simulink model "sig_kadet"  (R2022a)
settings: Solver=FixedStepAuto  StartTime=0.0  StopTime=10.0  FixedStep=framePeriod_s  RelTol=1e-3
undefined symbols (not defined in the file): Control, DiscIntNeverNeededParam, framePeriod_s
libraries: slpidlib x10, aerolibconvert2 x7, simulink_extras x2
(part 1 of 2)
settings Model: Creator=brian  LastModifiedBy=HP
settings SolverCC: AlgebraicLoopSolver=TrustRegion
settings OptimizationCC: DefaultParameterBehavior=Inlined  GainParamInheritBuiltInType=on  UseFloatMulNetSlope=on  DefaultUnderspecifiedDataType=single  InlineInvariantSignals=on  PassReuseOutputArgsAs=Individual arguments  ZeroExternalMemoryAtStartup=off  ZeroInternalMemoryAtStartup=off  NoFixptDivByZeroProtection=on  EfficientFloat2IntCast=on  LifeSpan=1  OptimizeBlockOrder=speed  DifferentSizesBufferReuse=on  EfficientTunableParamExpr=on
settings DebuggingCC: ParameterTunabilityLossMsg=error  UnconnectedInputMsg=warning  UnconnectedOutputMsg=warning  UnconnectedLineMsg=warning
settings HardwareCC: ProdBitPerPointer=32  ProdBitPerSizeT=32  ProdBitPerPtrDiffT=32  ProdLargestAtomicInteger=Long  ProdLargestAtomicFloat=Double  ProdWordSize=32  ProdLongLongMode=on  ProdHWDeviceType=NXP->Cortex-M4
settings ModelReferenceCC: ModelReferenceNumInstancesAllowed=Single
settings SFSimCC: SimParseCustomCode=off  MATLABDynamicMemAlloc=off
settings RTWCC: SystemTargetFile=ert.tlc  GenCodeOnly=on  TemplateMakefile=ert_default_tmf  RTWVerbose=off  Toolchain=Microsoft Visual C++ 2022 v17.0 | nmake (64-bit Windows)  BuildConfiguration=Faster Runs  TargetLang=C++  DLArmComputeVersion=19.05
settings CodeAppCC: ForceParamTrailComments=on  IgnoreCustomStorageClasses=off  OperatorAnnotations=on  SimulinkDataObjDesc=on  SFDataObjDesc=on  CustomSymbolStrGlobalVar=rt$N$M  CustomSymbolStrType=$N$M  CustomSymbolStrFcn=$N$M$F  CustomSymbolStrMacro=$N$M  InsertBlockDesc=on
settings ERTTargetCC: TargetLangStandard=C++03 (ISO)  IncludeMdlTerminateFcn=off  CombineSignalStateStructs=on  SuppressErrorStatus=on  SupportAbsoluteTime=off  CodeInterfacePackaging=C++ class  SupportNonFinite=off  SupportComplex=off  ERTHeaderFileRootName=autocode$E  ERTSourceFileRootName=autocode$E  InlinedParameterPlacement=NonHierarchical  RootIOFormat=Structure reference  ERTCustomFileTemplate=example_file_process.tlc  ERTFilePackagingFormat=Compact  ArrayContainerType=std::array

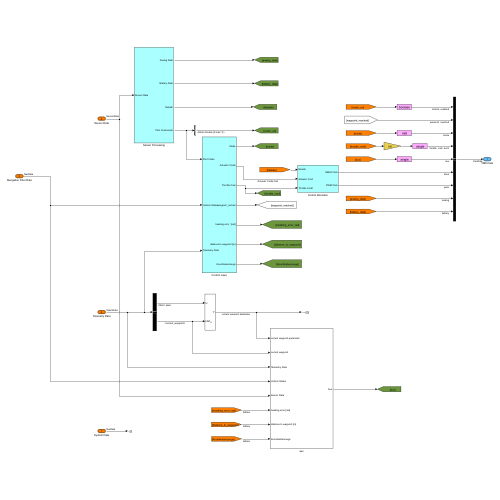
[thumbnail: Simulink's stored preview of the top-level diagram]
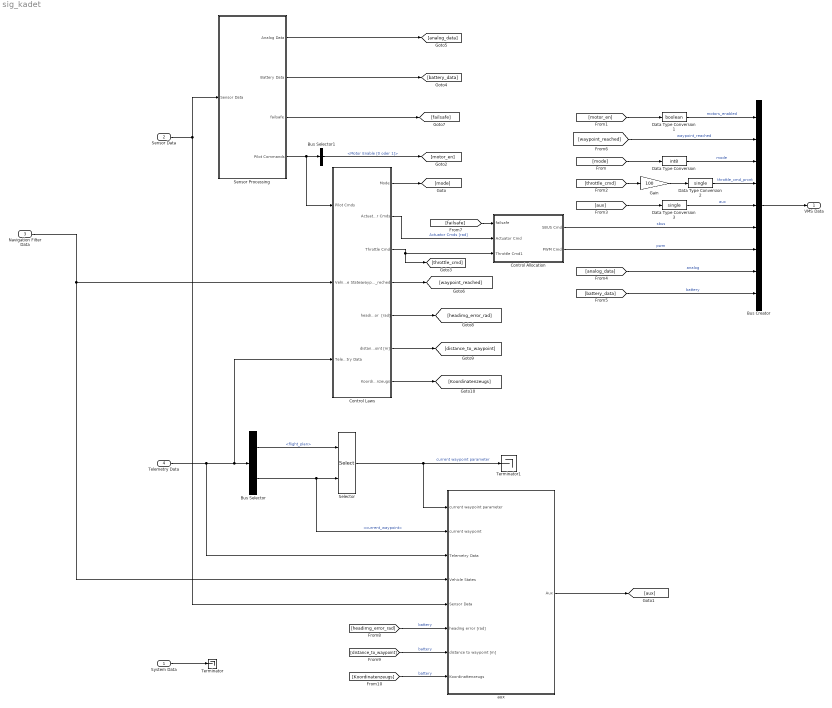
== system sig_kadet ==
  System Data : Inport  OutDataTypeStr=Bus: SysData  SampleTime=framePeriod_s  BusOutputAsStruct=on
  Sensor Data : Inport  Port=2  OutDataTypeStr=Bus: SensorData  SampleTime=framePeriod_s  BusOutputAsStruct=on
  Navigation Filter Data : Inport  Port=3  OutDataTypeStr=Bus: NavData  SampleTime=framePeriod_s  BusOutputAsStruct=on
  Telemetry Data : Inport  Port=4  OutDataTypeStr=Bus: TelemData  SampleTime=framePeriod_s  BusOutputAsStruct=on
  Bus Creator : BusCreator  Inputs=9
  Bus Selector : BusSelector  OutputSignals=flight_plan,current_waypoint
  Bus Selector1 : BusSelector  OutputSignals=Motor Enable [0 oder 1]
  Control Allocation : Subsystem
  Control Laws : Subsystem
  Data Type Conversion : DataTypeConversion  OutDataTypeStr=int8  SaturateOnIntegerOverflow=off  RndMeth=Floor
  Data Type Conversion1 : DataTypeConversion  OutDataTypeStr=boolean  SaturateOnIntegerOverflow=off  RndMeth=Floor
  Data Type Conversion2 : DataTypeConversion  OutDataTypeStr=single  SaturateOnIntegerOverflow=off  RndMeth=Floor
  Data Type Conversion3 : DataTypeConversion  OutDataTypeStr=single  SaturateOnIntegerOverflow=off  RndMeth=Floor
  Gain : Gain  Gain=100  OutDataTypeStr=single
  Selector : Selector  IndexMode=Zero-based  InputPortWidth=500  IndexOptions=Index vector (port)  Indices=[1 3]  OutputSizes=1
  Sensor Processing : Subsystem
  Terminator : Terminator
  Terminator1 : Terminator
  aux : Subsystem
  VMS Data : Outport  OutDataTypeStr=Bus: VmsData  SampleTime=framePeriod_s  BusOutputAsStruct=on
  wires:
  System Data/1 -> Terminator/1
  Sensor Data/1 -> aux/5(Sensor Data), Sensor Processing/1(Sensor Data)
  Telemetry Data/1 -> Control Laws/3(Telemetry Data), Bus Selector/1, aux/3(Telemetry Data)
  Navigation Filter Data/1 -> Control Laws/2(Vehicle States), aux/4(Vehicle States)
  Control Laws/1(Mode) -> [mode]
  [mode] -> Data Type Conversion/1
  Data Type Conversion/1 -> Bus Creator/3  "mode"
  Bus Selector1/1 -> [motor_en]  "<Motor Enable [0 oder 1]>"
  [motor_en] -> Data Type Conversion1/1
  Data Type Conversion1/1 -> Bus Creator/1  "motors_enabled"
  Control Laws/3(Throttle Cmd) -> [throttle_cmd], Control Allocation/3(Throttle Cmd1)
  [throttle_cmd] -> Gain/1
  Gain/1 -> Data Type Conversion2/1
  Data Type Conversion2/1 -> Bus Creator/4  "throttle_cmd_prcnt"
  [aux] -> Data Type Conversion3/1
  Data Type Conversion3/1 -> Bus Creator/5  "aux"
  Bus Creator/1 -> VMS Data/1
  Sensor Processing/4(Pilot Commands) -> Control Laws/1(Pilot Cmds), Bus Selector1/1
  Sensor Processing/2(Battery Data) -> [battery_data]
  Sensor Processing/1(Analog Data) -> [analog_data]
  [analog_data] -> Bus Creator/8  "analog"
  [battery_data] -> Bus Creator/9  "battery"
  Control Laws/2(Actuator Cmds) -> Control Allocation/2(Actuator Cmd)  "Actuator Cmds [rad]"
  Control Allocation/1(SBUS Cmd) -> Bus Creator/6  "sbus"
  Control Allocation/2(PWM Cmd) -> Bus Creator/7  "pwm"
  Bus Selector/1 -> Selector/1  "<flight_plan>"
  Bus Selector/2 -> aux/2(current waypoint), Selector/2  "<current_waypoint>"
  Selector/1 -> aux/1(current waypoint parameter), Terminator1/1  "current waypoint parameter"
  aux/1(Aux) -> [aux]
  Control Laws/4(waypoinr_reched) -> [waypoint_reached]
  [waypoint_reached] -> Bus Creator/2  "waypoint_reached"
  Sensor Processing/3(failsafe) -> [failsafe]
  [failsafe] -> Control Allocation/1(failsafe)
  Control Laws/5(heading error  [rad]) -> [headimg_error_rad]
  [headimg_error_rad] -> aux/6(heading error [rad])  "battery"
  Control Laws/6(distance to waypoint [m]) -> [distance_to_waypoint]
  [distance_to_waypoint] -> aux/7(distance to waypoint [m])  "battery"
  Control Laws/7(Koordinatenzeugs) -> [Koordinatenzeugs]
  [Koordinatenzeugs] -> aux/8(Koordinattenzeugs)  "battery"

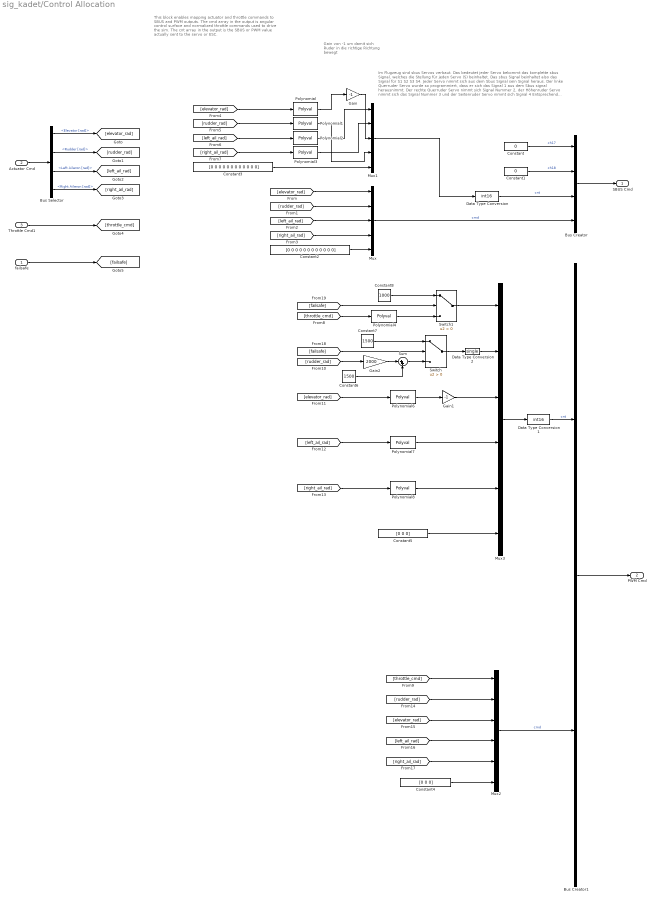
== system sig_kadet/Control Allocation ==
  note: Im Flugzeug sind sbus Servos verbaut. Das bedeutet jeder Servo bekommt das komplette sbus Signal, welches die Stellung für jeden Servo (S) beinhaltet. Das sbus Signal beinhaltet also das Signal für S1 S2 S3 S4. Jeder Servo nimmt sich aus dem Sbus Signal sein Signal heraus. Der linke Querruder Servo wurde so programmiert, dass er sich das Signal 1 aus dem Sbus signal herausnimmt. Der rechte Querruder Servo nimmt sich Signal Nummer 2, der Höhenruder Servo nimmt sich das Signal Nummer 3 und der Seitenruder Servo nimmt sich Signal 4
      |
      | Entsprechend der Programmierung der Servos muss das Sbus Signal aufgebaut werden, sodass z.B. sich der Höhenruderservo auch das Höhenrudersignal nimmt und nicht bspw, das von einem Querruder
  note: Gain von -1 um damit sich Ruder in die richtige Richtung bewegt
  note: This block enables mapping actuator and throttle commands
      | to SBUS and PWM outputs. The cmd array in the output
      | is angular control surface and normalized throttle commands
      | used to drive the sim. The cnt array in the output is the SBUS
      | or PWM value actually sent to the servo or ESC.
  failsafe : Inport
  Actuator Cmd : Inport  Port=2
  Throttle Cmd1 : Inport  Port=3
  Bus Creator : BusCreator  Inputs=4
  Bus Creator1 : BusCreator  Inputs=2
  Bus Selector : BusSelector  OutputSignals=Elevator [rad],Rudder [rad],Left Aileron [rad],Right Aileron [rad]
  Constant : Constant  Value=0  OutDataTypeStr=boolean
  Constant1 : Constant  Value=0  OutDataTypeStr=boolean
  Constant2 : Constant  Value=[0 0 0 0 0 0 0 0 0 0 0 0]  OutDataTypeStr=single
  Constant3 : Constant  Value=[0 0 0 0 0 0 0 0 0 0 0 0]  OutDataTypeStr=single
  Constant4 : Constant  Value=[0 0 0]  OutDataTypeStr=single
  Constant5 : Constant  Value=[0 0 0]  OutDataTypeStr=single
  Constant6 : Constant  Value=1500
  Constant7 : Constant  Value=1500
  Constant8 : Constant  Value=1000
  Data Type Conversion : DataTypeConversion  OutDataTypeStr=int16  SaturateOnIntegerOverflow=off  RndMeth=Floor
  Data Type Conversion1 : DataTypeConversion  OutDataTypeStr=int16  SaturateOnIntegerOverflow=off  RndMeth=Floor
  Data Type Conversion2 : DataTypeConversion  OutDataTypeStr=single  SaturateOnIntegerOverflow=off  RndMeth=Floor
  Gain : Gain  Gain=-1
  Gain1 : Gain  Gain=-1
  Gain2 : Gain  Gain=2000
  Mux : Mux  Inputs=5
  Mux1 : Mux  Inputs=5
  Mux2 : Mux  Inputs=6
  Mux3 : Mux  Inputs=6
  Polynomial : Polyval  Coefs=[1144.32190165984, 167.225360182927, 1558.74885501875, 1026.6382652891]
  Polynomial1 : Polyval  Coefs=[-930.322085258545, 148.612787752928, -1476.11502090935, 1006.01614399429]
  Polynomial2 : Polyval  Coefs=[1097.27825386315, 173.191562145482, 1642.60230905023, 1054.30469578325]
  Polynomial3 : Polyval  Coefs=[930.582953971947, 132.665450728095, 1620.14796233637, 1011.10438715363]
  Polynomial4 : Polyval  Coefs=[1000, 1000]
  Polynomial6 : Polyval  Coefs=[1144.32190165984, 167.225360182927, 1558.74885501875, 1026.6382652891]
  Polynomial7 : Polyval  Coefs=[1097.27825386315, 173.191562145482, 1642.60230905023, 1054.30469578325]
  Polynomial8 : Polyval  Coefs=[930.582953971947, 132.665450728095, 1620.14796233637, 1011.10438715363]
  Sum : Sum  Inputs=|++
  Switch : Switch  Criteria=u2 > Threshold  SaturateOnIntegerOverflow=off  InputSameDT=off
  Switch1 : Switch  Criteria=u2 > Threshold  SaturateOnIntegerOverflow=off  InputSameDT=off
  SBUS Cmd : Outport
  PWM Cmd : Outport  Port=2
  wires:
  Constant/1 -> Bus Creator/1  "ch17"
  Constant1/1 -> Bus Creator/2  "ch18"
  Bus Creator/1 -> SBUS Cmd/1
  Mux/1 -> Bus Creator/4  "cmd"
  Mux1/1 -> Data Type Conversion/1
  Actuator Cmd/1 -> Bus Selector/1
  Bus Selector/1 -> [elevator_rad]  "<Elevator [rad]>"
  Bus Selector/2 -> [rudder_rad]  "<Rudder [rad]>"
  Bus Selector/3 -> [left_ail_rad]  "<Left Aileron [rad]>"
  Bus Selector/4 -> [right_ail_rad]  "<Right Aileron [rad]>"
  [elevator_rad] -> Mux/1
  [rudder_rad] -> Mux/2
  [left_ail_rad] -> Mux/3
  [right_ail_rad] -> Mux/4
  Constant2/1 -> Mux/5
  Constant3/1 -> Mux1/5
  [right_ail_rad] -> Polynomial3/1
  [left_ail_rad] -> Polynomial2/1
  [rudder_rad] -> Polynomial1/1
  [elevator_rad] -> Polynomial/1
  Data Type Conversion/1 -> Bus Creator/3  "cnt"
  Polynomial/1 -> Gain/1
  Polynomial1/1 -> Mux1/4
  Polynomial2/1 -> Mux1/1
  Polynomial3/1 -> Mux1/2
  Bus Creator1/1 -> PWM Cmd/1
  Mux2/1 -> Bus Creator1/2  "cmd"
  Constant4/1 -> Mux2/6
  [throttle_cmd] -> Polynomial4/1
  Polynomial4/1 -> Switch1/3
  Constant5/1 -> Mux3/6
  Data Type Conversion1/1 -> Bus Creator1/1  "cnt"
  Gain/1 -> Mux1/3
  Throttle Cmd1/1 -> [throttle_cmd]
  [throttle_cmd] -> Mux2/1
  [elevator_rad] -> Mux2/3
  Mux3/1 -> Data Type Conversion1/1
  [rudder_rad] -> Gain2/1
  Polynomial6/1 -> Gain1/1
  [elevator_rad] -> Polynomial6/1
  Gain1/1 -> Mux3/3
  [left_ail_rad] -> Polynomial7/1
  [right_ail_rad] -> Polynomial8/1
  Polynomial7/1 -> Mux3/4
  Polynomial8/1 -> Mux3/5
  [right_ail_rad] -> Mux2/5
  [left_ail_rad] -> Mux2/4
  [rudder_rad] -> Mux2/2
  Constant6/1 -> Sum/2
  Sum/1 -> Switch/3
  Data Type Conversion2/1 -> Mux3/2
  Gain2/1 -> Sum/1
  failsafe/1 -> [failsafe]
  Switch/1 -> Data Type Conversion2/1
  [failsafe] -> Switch/2
  Constant7/1 -> Switch/1
  Switch1/1 -> Mux3/1
  [failsafe] -> Switch1/2
  Constant8/1 -> Switch1/1

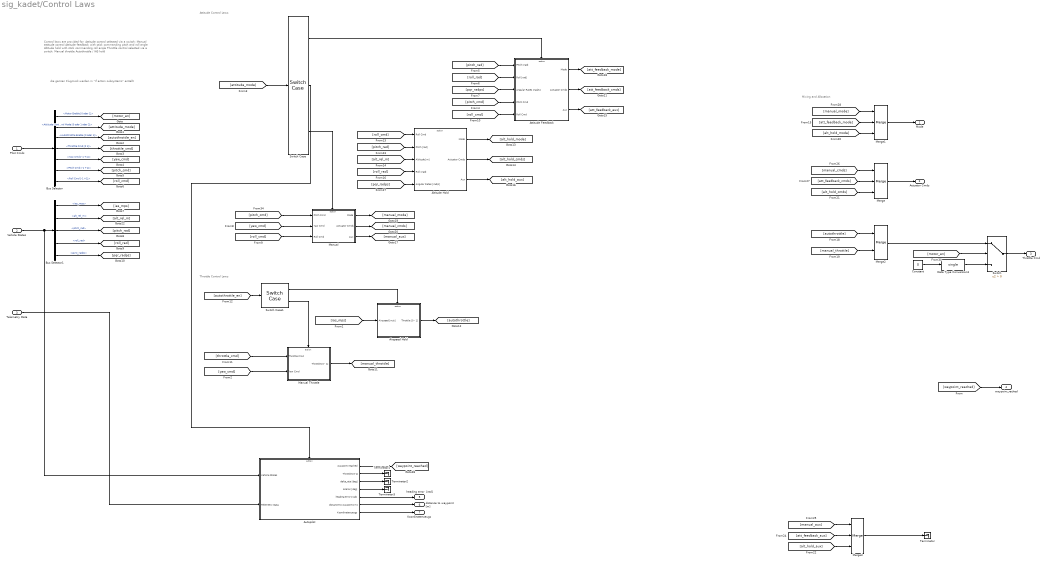
== system sig_kadet/Control Laws ==
  note: die ganzen Flugmodi werden in "if action subsystems"
      | erstellt
  note: Control laws are provided for:
      | Attitude control selected via a switch:
      | Manual attitude control
      | Attitude feedback with stick commanding pitch and roll angle
      | Altitude hold with stick commanding roll angle
      | Throttle control selected via a switch:
      | Manual throttle
      | Autothrottle / IAS hold
  note: Throttle Control Laws
  note: Attitude Control Laws
  note: Mixing and Allocation
  Pilot Cmds : Inport
  Vehicle States : Inport  Port=2
  Telemetry Data : Inport  Port=3
  Airspeed Hold : Subsystem  TreatAsAtomicUnit=on
  Altitude Hold : Subsystem  TreatAsAtomicUnit=on
  Attitude Feedback : Subsystem  TreatAsAtomicUnit=on
  Autopilot : Subsystem  TreatAsAtomicUnit=on
  Bus Selector : BusSelector  OutputSignals=Motor Enable [0 oder 1],Attitude Control Mode [0 oder 1 oder 2],Autothrottle Enable [0 oder 1],Throttle Cmd [0 1],Yaw Cmd [-1 +1],Pitch Cmd [-1 +1],Roll Cmd [-1 +1]
  Bus Selector1 : BusSelector  OutputSignals=ias_mps,alt_rel_m,pitch_rad,roll_rad,gyro_radps
  Constant : Constant  Value=0
  Data Type Conversion3 : DataTypeConversion  OutDataTypeStr=single  SaturateOnIntegerOverflow=off  RndMeth=Floor
  Manual : Subsystem  TreatAsAtomicUnit=on
  Manual Throttle : Subsystem  TreatAsAtomicUnit=on
  Merge : Merge  Inputs=3
  Merge1 : Merge  Inputs=3
  Merge2 : Merge
  Merge3 : Merge  Inputs=3
  Switch : Switch  Criteria=u2 > Threshold  OutDataTypeStr=single  SaturateOnIntegerOverflow=off  InputSameDT=off
  Switch Case : SwitchCase  CaseConditions={1, 2}
  Switch Case1 : SwitchCase
  Terminator{,1..3} (4 alike) : Terminator
  Mode : Outport
  Actuator Cmds : Outport  Port=2
  Throttle Cmd : Outport  Port=3
  waypoinr_reched : Outport  Port=4
  heading error  [rad] : Outport  Port=5
  distance to waypoint [m] : Outport  Port=6
  Koordinatenzeugs : Outport  Port=7
  wires:
  Pilot Cmds/1 -> Bus Selector/1
  Bus Selector/1 -> [motor_en]  "<Motor Enable [0 oder 1]>"
  Bus Selector/2 -> [attitude_mode]  "<Attitude Control Mode [0 oder 1 oder 2]>"
  Bus Selector/3 -> [autothrottle_en]  "<Autothrottle Enable [0 oder 1]>"
  Bus Selector/4 -> [throttle_cmd]  "<Throttle Cmd [0 1]>"
  Bus Selector/5 -> [yaw_cmd]  "<Yaw Cmd [-1 +1]>"
  Bus Selector/6 -> [pitch_cmd]  "<Pitch Cmd [-1 +1]>"
  Bus Selector/7 -> [roll_cmd]  "<Roll Cmd [-1 +1]>"
  Vehicle States/1 -> Autopilot/1(Vehicle States), Bus Selector1/1
  Bus Selector1/1 -> [ias_mps]  "<ias_mps>"
  Bus Selector1/3 -> [pitch_rad]  "<pitch_rad>"
  Bus Selector1/4 -> [roll_rad]  "<roll_rad>"
  Bus Selector1/5 -> [pqr_radps]  "<gyro_radps>"
  Airspeed Hold/1(Throttle [0 - 1]) -> [autothrottle]
  [ias_mps] -> Airspeed Hold/1(Airspeed [m/s])
  [autothrottle_en] -> Switch Case1/1
  [throttle_cmd] -> Manual Throttle/1(Throttle Cmd)
  Switch Case1/1 -> Airspeed Hold/Action
  Switch Case1/2 -> Manual Throttle/Action
  Manual Throttle/1(Throttle [0 - 1]) -> [manual_throttle]
  Manual/1(Mode) -> [manual_mode]
  [pqr_radps] -> Attitude Feedback/3(Angular Rates [rad/s])
  [pqr_radps] -> Altitude Hold/5(Angular Rates [rad/s])
  Altitude Hold/3(Aux) -> [alt_hold_aux]
  Altitude Hold/1(Mode) -> [alt_hold_mode]
  Manual/3(Aux) -> [manual_aux]
  [roll_cmd] -> Altitude Hold/1(Roll Cmd)
  Attitude Feedback/2(Actuator Cmds) -> [att_feedback_cmds]
  Switch Case/3 -> Manual/Action
  Manual/2(Actuator Cmds) -> [manual_cmds]
  Attitude Feedback/1(Mode) -> [att_feedback_mode]
  [roll_rad] -> Attitude Feedback/2(Roll [rad])
  [pitch_rad] -> Attitude Feedback/1(Pitch [rad])
  [alt_rel_m] -> Altitude Hold/3(Altitude [m])
  Switch Case/1 -> Attitude Feedback/Action
  Altitude Hold/2(Actuator Cmds) -> [alt_hold_cmds]
  [roll_rad] -> Altitude Hold/4(Roll [rad])
  [pitch_rad] -> Altitude Hold/2(Pitch [rad])
  Attitude Feedback/3(Aux) -> [att_feedback_aux]
  Switch Case/2 -> Autopilot/Action
  [attitude_mode] -> Switch Case/1
  [yaw_cmd] -> Manual/2(Yaw Cmd)
  [roll_cmd] -> Manual/3(Roll Cmd)
  [pitch_cmd] -> Attitude Feedback/4(Pitch Cmd)
  [roll_cmd] -> Attitude Feedback/5(Roll Cmd)
  Bus Selector1/2 -> [alt_rel_m]  "<alt_rel_m>"
  Merge3/1 -> Terminator/1
  [att_feedback_aux] -> Merge3/2
  [alt_hold_aux] -> Merge3/3
  [manual_aux] -> Merge3/1
  [att_feedback_cmds] -> Merge/2
  [alt_hold_cmds] -> Merge/3
  [alt_hold_mode] -> Merge1/3
  [autothrottle] -> Merge2/1
  Merge1/1 -> Mode/1
  [manual_mode] -> Merge1/1
  [manual_cmds] -> Merge/1
  [att_feedback_mode] -> Merge1/2
  Merge/1 -> Actuator Cmds/1
  [manual_throttle] -> Merge2/2
  Merge2/1 -> Switch/1
  [motor_en] -> Switch/2
  Constant/1 -> Data Type Conversion3/1
  Switch/1 -> Throttle Cmd/1
  [pitch_cmd] -> Manual/1(Pitch Cmd)
  Data Type Conversion3/1 -> Switch/3
  [yaw_cmd] -> Manual Throttle/2(Yaw Cmd)
  Telemetry Data/1 -> Autopilot/2(Telemetry Data)
  Autopilot/1(waypoint reached) -> [waypoint_reached]
  [waypoint_reached] -> waypoinr_reched/1
  Autopilot/2(Throttle [0-1]) -> Terminator1/1
  Autopilot/3(delta_eta [deg]) -> Terminator2/1
  Autopilot/4(aileron [deg]) -> Terminator3/1
  Autopilot/5(heading error [rad]) -> heading error  [rad]/1
  Autopilot/6(distance to waypoint [m]) -> distance to waypoint [m]/1
  Autopilot/7(Koordinatenzeugs) -> Koordinatenzeugs/1

== system sig_kadet/Sensor Processing ==
  Sensor Data : Inport
  Analog Input Mapping : Subsystem
  Battery Data and State Estimation : Subsystem
  Bus Selector : BusSelector  OutputSignals=inceptor,adc,power_module,inceptor.failsafe
  Pilot Stick Mapping : Subsystem
  Analog Data : Outport
  Battery Data : Outport  Port=2
  failsafe : Outport  Port=3
  Pilot Commands : Outport  Port=4
  wires:
  Pilot Stick Mapping/1(Pilot Commands) -> Pilot Commands/1
  Sensor Data/1 -> Bus Selector/1
  Bus Selector/1 -> Pilot Stick Mapping/1(Inceptors)  "<inceptor>"
  Bus Selector/3 -> Battery Data and State Estimation/1(Power Module Data)  "<power_module>"
  Analog Input Mapping/1(Analog Data) -> Analog Data/1
  Battery Data and State Estimation/1(Battery Data) -> Battery Data/1
  Bus Selector/2 -> Analog Input Mapping/1(ADC)  "<adc>"
  Bus Selector/4 -> failsafe/1  "<failsafe>"

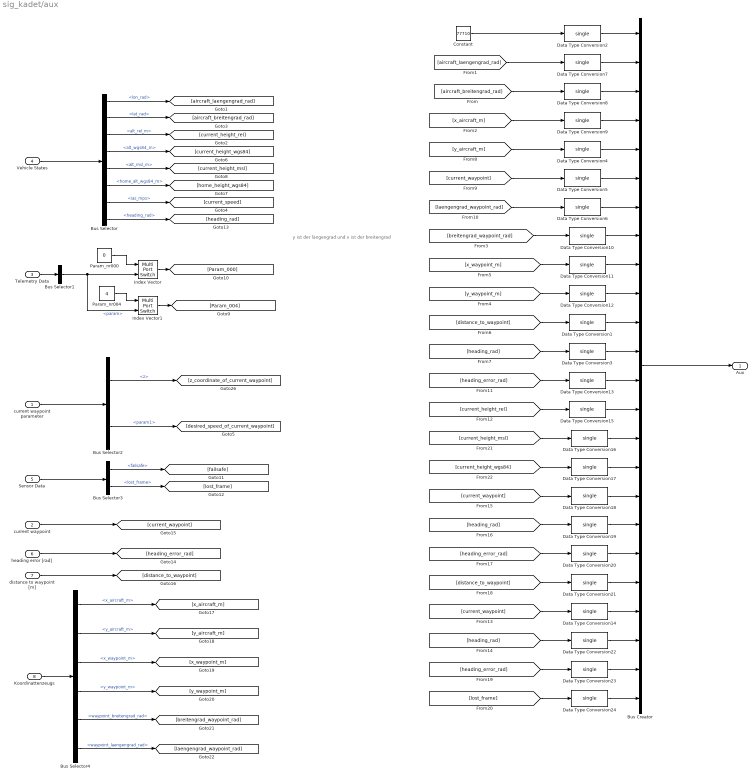
== system sig_kadet/aux ==
  note: y ist der längengrad und x ist der breitengrad
  current waypoint parameter : Inport
  current waypoint : Inport  Port=2
  Telemetry Data : Inport  Port=3
  Vehicle States : Inport  Port=4
  Sensor Data : Inport  Port=5
  heading error [rad] : Inport  Port=6
  distance to waypoint [m] : Inport  Port=7
  Koordinattenzeugs : Inport  Port=8
  Bus Creator : BusCreator  Inputs=24
  Bus Selector : BusSelector  OutputSignals=lon_rad,lat_rad,alt_rel_m,alt_wgs84_m,alt_msl_m,home_alt_wgs84_m,ias_mps,heading_rad
  Bus Selector1 : BusSelector  OutputSignals=param
  Bus Selector2 : BusSelector  OutputSignals=z,param1
  Bus Selector3 : BusSelector  OutputSignals=inceptor.failsafe,inceptor.lost_frame
  Bus Selector4 : BusSelector  OutputSignals=x_aircraft_m,y_aircraft_m,x_waypoint_m,y_waypoint_m,waypoint_breitengrad_rad,waypoint_laengengrad_rad
  Constant : Constant  Value=77710
  Data Type Conversion{1..24} (24 alike) : DataTypeConversion  OutDataTypeStr=single  SaturateOnIntegerOverflow=off  RndMeth=Floor
  Index Vector : MultiPortSwitch  DataPortOrder=Zero-based contiguous  Inputs=1  zeroidx=on  SaturateOnIntegerOverflow=off  InputSameDT=off
  Index Vector1 : MultiPortSwitch  DataPortOrder=Zero-based contiguous  Inputs=1  zeroidx=on  SaturateOnIntegerOverflow=off  InputSameDT=off
  Param_nr000 : Constant  Value=0
  Param_nr004 : Constant  Value=4
  Aux : Outport
  wires:
  Data Type Conversion14/1 -> Bus Creator/21
  Data Type Conversion11/1 -> Bus Creator/9
  [y_waypoint_m] -> Data Type Conversion12/1
  Bus Creator/1 -> Aux/1
  [x_waypoint_m] -> Data Type Conversion11/1
  Data Type Conversion12/1 -> Bus Creator/10
  [breitengrad_waypoint_rad] -> Data Type Conversion10/1
  [aircraft_laengengrad_rad] -> Data Type Conversion7/1
  [aircraft_breitengrad_rad] -> Data Type Conversion8/1
  Data Type Conversion7/1 -> Bus Creator/2
  Data Type Conversion10/1 -> Bus Creator/8
  [x_aircraft_m] -> Data Type Conversion9/1
  Data Type Conversion8/1 -> Bus Creator/3
  Data Type Conversion9/1 -> Bus Creator/4
  Bus Selector2/1 -> [z_coordinate_of_current_waypoint]  "<z>"
  current waypoint parameter/1 -> Bus Selector2/1
  Vehicle States/1 -> Bus Selector/1
  Bus Selector/7 -> [current_speed]  "<ias_mps>"
  Bus Selector/2 -> [aircraft_breitengrad_rad]  "<lat_rad>"
  Bus Selector/1 -> [aircraft_laengengrad_rad]  "<lon_rad>"
  Bus Selector/3 -> [current_height_rel]  "<alt_rel_m>"
  [distance_to_waypoint] -> Data Type Conversion1/1
  Data Type Conversion1/1 -> Bus Creator/11
  Constant/1 -> Data Type Conversion2/1
  Data Type Conversion2/1 -> Bus Creator/1
  Bus Selector2/2 -> [desired_speed_of_current_waypoint]  "<param1>"
  Data Type Conversion3/1 -> Bus Creator/12
  [heading_rad] -> Data Type Conversion3/1
  Bus Selector/4 -> [current_height_wgs84]  "<alt_wgs84_m>"
  Bus Selector/6 -> [home_height_wgs84]  "<home_alt_wgs84_m>"
  Bus Selector/5 -> [current_height_msl]  "<alt_msl_m>"
  Data Type Conversion4/1 -> Bus Creator/5
  [y_aircraft_m] -> Data Type Conversion4/1
  [current_waypoint] -> Data Type Conversion5/1
  [laengengrad_waypoint_rad] -> Data Type Conversion6/1
  Data Type Conversion5/1 -> Bus Creator/6
  Data Type Conversion6/1 -> Bus Creator/7
  Bus Selector1/1 -> Index Vector1/2, Index Vector/2  "<param>"
  Param_nr000/1 -> Index Vector/1
  Param_nr004/1 -> Index Vector1/1
  Index Vector/1 -> [Param_000]
  Index Vector1/1 -> [Param_004]
  [current_height_rel] -> Data Type Conversion15/1
  Data Type Conversion15/1 -> Bus Creator/14
  Data Type Conversion13/1 -> Bus Creator/13
  [heading_error_rad] -> Data Type Conversion13/1
  Telemetry Data/1 -> Bus Selector1/1
  Sensor Data/1 -> Bus Selector3/1
  Bus Selector3/1 -> [failsafe]  "<failsafe>"
  [current_height_msl] -> Data Type Conversion16/1
  Data Type Conversion16/1 -> Bus Creator/15
  Bus Selector3/2 -> [lost_frame]  "<lost_frame>"
  Data Type Conversion17/1 -> Bus Creator/16
  Bus Selector/8 -> [heading_rad]  "<heading_rad>"
  [current_waypoint] -> Data Type Conversion18/1
  Data Type Conversion18/1 -> Bus Creator/17
  heading error [rad]/1 -> [heading_error_rad]
  current waypoint/1 -> [current_waypoint]
  [heading_error_rad] -> Data Type Conversion20/1
  [heading_rad] -> Data Type Conversion19/1
  Data Type Conversion19/1 -> Bus Creator/18
  Data Type Conversion20/1 -> Bus Creator/19
  distance to waypoint [m]/1 -> [distance_to_waypoint]
  [distance_to_waypoint] -> Data Type Conversion21/1
  Data Type Conversion21/1 -> Bus Creator/20
  Koordinattenzeugs/1 -> Bus Selector4/1
  Bus Selector4/1 -> [x_aircraft_m]  "<x_aircraft_m>"
  Bus Selector4/2 -> [y_aircraft_m]  "<y_aircraft_m>"
  Bus Selector4/3 -> [x_waypoint_m]  "<x_waypoint_m>"
  Bus Selector4/4 -> [y_waypoint_m]  "<y_waypoint_m>"
  Bus Selector4/5 -> [breitengrad_waypoint_rad]  "<waypoint_breitengrad_rad>"
  Bus Selector4/6 -> [laengengrad_waypoint_rad]  "<waypoint_laengengrad_rad>"
  [lost_frame] -> Data Type Conversion24/1
  [heading_rad] -> Data Type Conversion22/1
  [heading_error_rad] -> Data Type Conversion23/1
  [current_waypoint] -> Data Type Conversion14/1
  Data Type Conversion22/1 -> Bus Creator/22
  Data Type Conversion23/1 -> Bus Creator/23
  Data Type Conversion24/1 -> Bus Creator/24
  [current_height_wgs84] -> Data Type Conversion17/1

== system sig_kadet/Control Laws/Airspeed Hold ==
  Airspeed [m/s] : Inport
  Action Port : ActionPort  InitializeStates=reset  ActionPortLabel=case [ 1 ]:
  Constant1 : Constant  Value=Control.Airspeed.ref_mps  OutDataTypeStr=single
  Constant2 : Constant  Value=framePeriod_s  OutDataTypeStr=single
  PID Controller : slpidlib/PID Controller  Controller=PID  Form=Parallel  TimeDomain=Discrete-time  UseExternalTs=on  SampleTime=-1  IntegratorMethod=Forward Euler  FilterMethod=Forward Euler  ControllerParametersSource=internal  P=Control.Airspeed.p  I=Control.Airspeed.i  D=0  UseFilter=off  N=100  TunerSelectOption=Transfer Function Based (PID Tuner App)  ZeroCross=off  InitialConditionSource=internal  InitialConditionForIntegrator=0  InitialConditionForFilter=0  DifferentiatorICPrevScaledInput=0  ExternalReset=none  TrackingMode=off  Kt=1  LimitOutput=on  SatLimitsSource=internal  UpperSaturationLimit=Control.pla_lim_max  LowerSaturationLimit=Control.pla_lim_min  LinearizeAsGain=on  AntiWindupMode=clamping  Kb=1  PGainOutDataTypeStr=single  PProdOutDataTypeStr=single  POutMin=[]  POutMax=[]  IGainOutDataTypeStr=single  IProdOutDataTypeStr=single  IOutMin=[]  IOutMax=[]  DGainOutDataTypeStr=single  DProdOutDataTypeStr=single  DOutMin=[]  DOutMax=[]  NOutMin=[]  NOutMax=[]  SumOutDataTypeStr=single  SumOutMin=[]  SumOutMax=[]  SaturationOutDataTypeStr=single  SaturationOutMin=[]  SaturationOutMax=[]  PParamMin=[]  PParamMax=[]  IParamMin=[]  IParamMax=[]  DParamMin=[]  DParamMax=[]  NParamMin=[]  NParamMax=[]  KbParamMin=[]  KbParamMax=[]  KtParamMin=[]  KtParamMax=[]  KbOutMin=[]  KbOutMax=[]  KtOutMin=[]  KtOutMax=[]  IntegratorOutMin=[]  IntegratorOutMax=[]  FilterOutMin=[]  FilterOutMax=[]  SumI1OutMin=[]  SumI1OutMax=[]  SumI2OutMin=[]  SumI2OutMax=[]  SumI3OutMin=[]  SumI3OutMax=[]  SumI4OutMin=[]  SumI4OutMax=[]  SumDOutMin=[]  SumDOutMax=[]  DifferentiatorOutMin=[]  DifferentiatorOutMax=[]  FilterDiffOutCoefMin=[]  FilterDiffOutCoefMax=[]  ReciprocalOutMin=[]  ReciprocalOutMax=[]  SumDenOutMin=[]  SumDenOutMax=[]  SumNumOutMin=[]  SumNumOutMax=[]  DivideOutMin=[]  DivideOutMax=[]  UdiffTsProdOutMin=[]  UdiffTsProdOutMax=[]  NTsProdOutMin=[]  NTsProdOutMax=[]  UintegralTsProdOutMin=[]  UintegralTsProdOutMax=[]  UngainTsProdOutMin=[]  UngainTsProdOutMax=[]  IntegratorContinuousStateAttributes=''  IntegratorStateMustResolveToSignalObject=off  IntegratorRTWStateStorageClass=Auto  FilterContinuousStateAttributes=''  FilterStateMustResolveToSignalObject=off  FilterRTWStateStorageClass=Auto  ParallelPVariant=InternalParameters  IdealPVariant=Disabled  IVariant=InternalParameters  DVariant=InternalParameters  IntegratorVariant=Discrete  SatVariant=Enabled  AWVariant=DiscClampingParallel  PCopyVariant=Disabled  TRVariant=Disabled  FdbkBlocksVariant=Forward  IdealPFdbkVariant=Disabled  SatFdbkVariant=Disabled  DerivativeFilterVariant=Differentiator  NVariant=Passthrough  NCopyVariant=Disabled_SignalSpec  FilterICVariant=InternalICsDifferentiator  IntegratorICVariant=InternalICs  ExternalResetVariant=Disabled  TRSumVariant=Passthrough  SumFdbkVariant=Disabled  SumVariant=Sum_PID  TsampFilterVariant=ExternalTs  TsampNgainVariant=Passthrough  TsampIntegralVariant=ExternalTs  ExternalSaturationOutDataTypeStr=Inherit: Same as second input
  Subtract : Sum  Inputs=+-  AccumDataTypeStr=single
  Throttle [0 - 1] : Outport
  wires:
  PID Controller/1 -> Throttle [0 - 1]/1  "Throttle [0 - 1]"
  Subtract/1 -> PID Controller/1
  Constant2/1 -> PID Controller/2
  Airspeed [m/s]/1 -> Subtract/2
  Constant1/1 -> Subtract/1

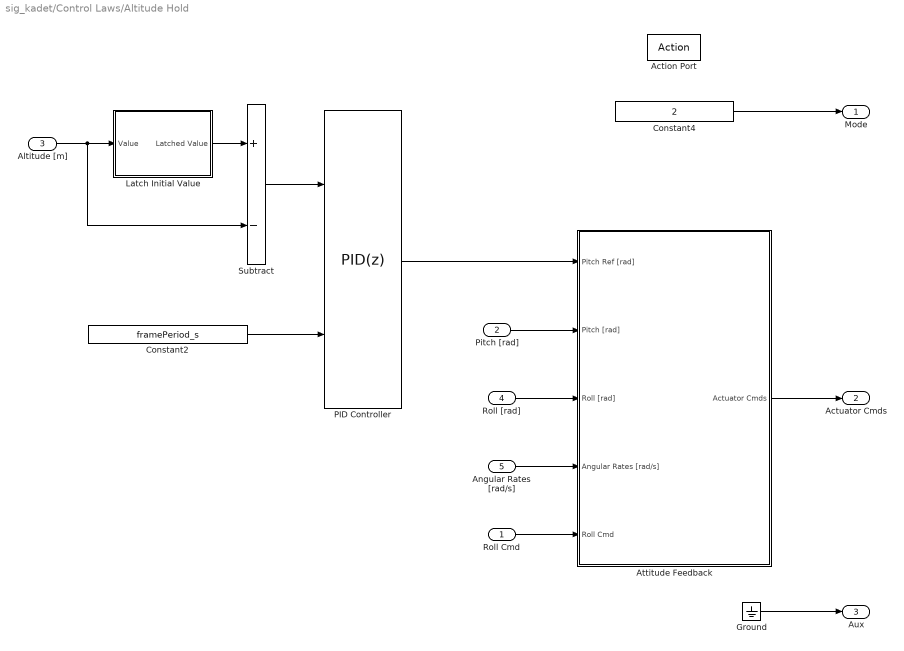
== system sig_kadet/Control Laws/Altitude Hold ==
  Roll Cmd : Inport
  Pitch [rad] : Inport  Port=2
  Altitude [m] : Inport  Port=3
  Roll [rad] : Inport  Port=4
  Angular Rates [rad/s] : Inport  Port=5
  Action Port : ActionPort  InitializeStates=reset
  Attitude Feedback : Subsystem  TreatAsAtomicUnit=on
  Constant2 : Constant  Value=framePeriod_s  OutDataTypeStr=single
  Constant4 : Constant  Value=2  OutDataTypeStr=int8
  Ground : Ground
  Latch Initial Value : Subsystem
  PID Controller : slpidlib/PID Controller  Controller=PID  Form=Parallel  TimeDomain=Discrete-time  UseExternalTs=on  SampleTime=-1  IntegratorMethod=Forward Euler  FilterMethod=Forward Euler  ControllerParametersSource=internal  P=Control.Altitude.p  I=Control.Altitude.i  D=0  UseFilter=off  N=100  TunerSelectOption=Transfer Function Based (PID Tuner App)  ZeroCross=off  InitialConditionSource=internal  InitialConditionForIntegrator=0  InitialConditionForFilter=0  DifferentiatorICPrevScaledInput=0  ExternalReset=none  TrackingMode=off  Kt=1  LimitOutput=on  SatLimitsSource=internal  UpperSaturationLimit=deg2rad(Control.pitch_lim_deg)  LowerSaturationLimit=-deg2rad(Control.pitch_lim_deg)  LinearizeAsGain=on  AntiWindupMode=clamping  Kb=1  PGainOutDataTypeStr=single  PProdOutDataTypeStr=single  POutMin=[]  POutMax=[]  IGainOutDataTypeStr=single  IProdOutDataTypeStr=single  IOutMin=[]  IOutMax=[]  DGainOutDataTypeStr=single  DProdOutDataTypeStr=single  DOutMin=[]  DOutMax=[]  NOutMin=[]  NOutMax=[]  SumOutDataTypeStr=single  SumOutMin=[]  SumOutMax=[]  SaturationOutDataTypeStr=single  SaturationOutMin=[]  SaturationOutMax=[]  PParamMin=[]  PParamMax=[]  IParamMin=[]  IParamMax=[]  DParamMin=[]  DParamMax=[]  NParamMin=[]  NParamMax=[]  KbParamMin=[]  KbParamMax=[]  KtParamMin=[]  KtParamMax=[]  KbOutMin=[]  KbOutMax=[]  KtOutMin=[]  KtOutMax=[]  IntegratorOutMin=[]  IntegratorOutMax=[]  FilterOutMin=[]  FilterOutMax=[]  SumI1OutMin=[]  SumI1OutMax=[]  SumI2OutMin=[]  SumI2OutMax=[]  SumI3OutMin=[]  SumI3OutMax=[]  SumI4OutMin=[]  SumI4OutMax=[]  SumDOutMin=[]  SumDOutMax=[]  DifferentiatorOutMin=[]  DifferentiatorOutMax=[]  FilterDiffOutCoefMin=[]  FilterDiffOutCoefMax=[]  ReciprocalOutMin=[]  ReciprocalOutMax=[]  SumDenOutMin=[]  SumDenOutMax=[]  SumNumOutMin=[]  SumNumOutMax=[]  DivideOutMin=[]  DivideOutMax=[]  UdiffTsProdOutMin=[]  UdiffTsProdOutMax=[]  NTsProdOutMin=[]  NTsProdOutMax=[]  UintegralTsProdOutMin=[]  UintegralTsProdOutMax=[]  UngainTsProdOutMin=[]  UngainTsProdOutMax=[]  IntegratorContinuousStateAttributes=''  IntegratorStateMustResolveToSignalObject=off  IntegratorRTWStateStorageClass=Auto  FilterContinuousStateAttributes=''  FilterStateMustResolveToSignalObject=off  FilterRTWStateStorageClass=Auto  ParallelPVariant=InternalParameters  IdealPVariant=Disabled  IVariant=InternalParameters  DVariant=InternalParameters  IntegratorVariant=Discrete  SatVariant=Enabled  AWVariant=DiscClampingParallel  PCopyVariant=Disabled  TRVariant=Disabled  FdbkBlocksVariant=Forward  IdealPFdbkVariant=Disabled  SatFdbkVariant=Disabled  DerivativeFilterVariant=Differentiator  NVariant=Passthrough  NCopyVariant=Disabled_SignalSpec  FilterICVariant=InternalICsDifferentiator  IntegratorICVariant=InternalICs  ExternalResetVariant=Disabled  TRSumVariant=Passthrough  SumFdbkVariant=Disabled  SumVariant=Sum_PID  TsampFilterVariant=ExternalTs  TsampNgainVariant=Passthrough  TsampIntegralVariant=ExternalTs  ExternalSaturationOutDataTypeStr=Inherit: Same as second input
  Subtract : Sum  Inputs=+-
  Mode : Outport
  Actuator Cmds : Outport  Port=2
  Aux : Outport  Port=3
  wires:
  Constant4/1 -> Mode/1
  Angular Rates [rad/s]/1 -> Attitude Feedback/4(Angular Rates [rad/s])
  Roll [rad]/1 -> Attitude Feedback/3(Roll [rad])
  Roll Cmd/1 -> Attitude Feedback/5(Roll Cmd)
  Attitude Feedback/1(Actuator Cmds) -> Actuator Cmds/1
  Altitude [m]/1 -> Subtract/2, Latch Initial Value/1(Value)
  Constant2/1 -> PID Controller/2
  Latch Initial Value/1(Latched Value) -> Subtract/1
  Subtract/1 -> PID Controller/1
  Ground/1 -> Aux/1
  Pitch [rad]/1 -> Attitude Feedback/2(Pitch [rad])
  PID Controller/1 -> Attitude Feedback/1(Pitch Ref [rad])

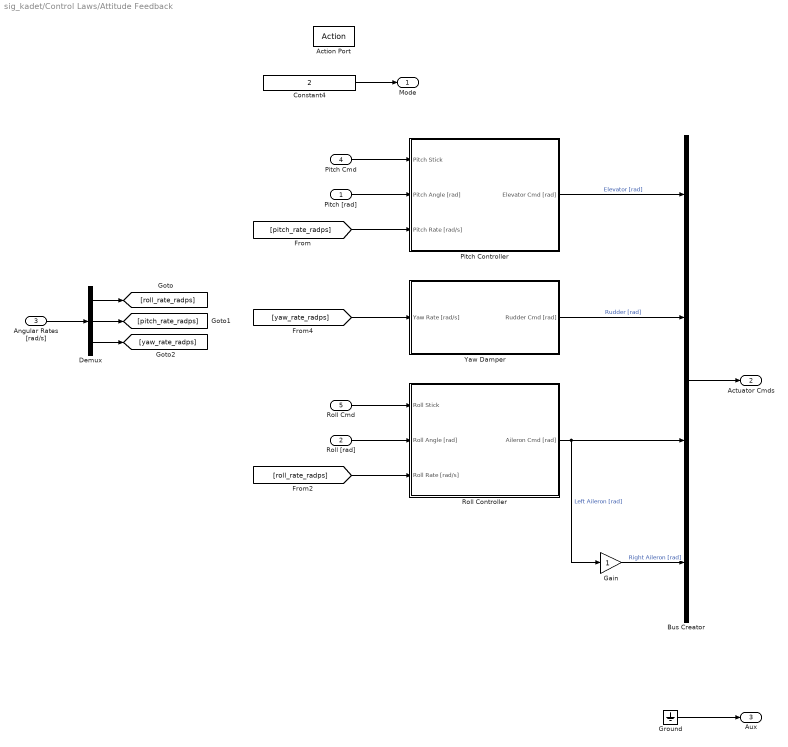
== system sig_kadet/Control Laws/Attitude Feedback ==
  Pitch [rad] : Inport
  Roll [rad] : Inport  Port=2
  Angular Rates [rad/s] : Inport  Port=3
  Pitch Cmd : Inport  Port=4
  Roll Cmd : Inport  Port=5
  Action Port : ActionPort  InitializeStates=reset  ActionPortLabel=case [ 1 ]:
  Bus Creator : BusCreator  Inputs=4
  Constant4 : Constant  Value=2  OutDataTypeStr=int8
  Demux : Demux  Outputs=3
  Gain : Gain
  Ground : Ground
  Pitch Controller : Subsystem
  Roll Controller : Subsystem
  Yaw Damper : Subsystem
  Mode : Outport
  Actuator Cmds : Outport  Port=2
  Aux : Outport  Port=3
  wires:
  Constant4/1 -> Mode/1
  Pitch [rad]/1 -> Pitch Controller/2(Pitch Angle [rad])
  Angular Rates [rad/s]/1 -> Demux/1
  Demux/1 -> [roll_rate_radps]
  Demux/3 -> [yaw_rate_radps]
  Demux/2 -> [pitch_rate_radps]
  [pitch_rate_radps] -> Pitch Controller/3(Pitch Rate [rad/s])
  Pitch Cmd/1 -> Pitch Controller/1(Pitch Stick)
  Pitch Controller/1(Elevator Cmd [rad]) -> Bus Creator/1  "Elevator [rad]"
  Bus Creator/1 -> Actuator Cmds/1
  Gain/1 -> Bus Creator/4  "Right Aileron [rad]"
  Roll Controller/1(Aileron Cmd [rad]) -> Gain/1, Bus Creator/3  "Left Aileron [rad]"
  Yaw Damper/1(Rudder Cmd [rad]) -> Bus Creator/2  "Rudder [rad]"
  Roll [rad]/1 -> Roll Controller/2(Roll Angle [rad])
  [roll_rate_radps] -> Roll Controller/3(Roll Rate [rad/s])
  Roll Cmd/1 -> Roll Controller/1(Roll Stick)
  [yaw_rate_radps] -> Yaw Damper/1(Yaw Rate [rad/s])
  Ground/1 -> Aux/1

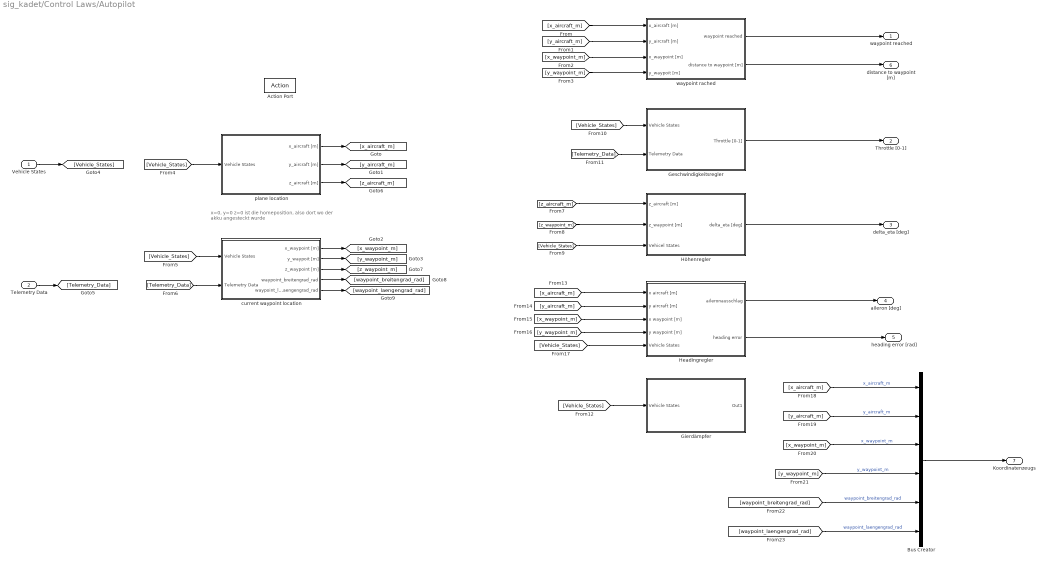
== system sig_kadet/Control Laws/Autopilot ==
  note: x=0, y=0 z=0 ist die homeposition, also
      | dort wo der akku angesteckt wurde
  Vehicle States : Inport
  Telemetry Data : Inport  Port=2
  Action Port : ActionPort  ActionPortLabel=case [ 2 ]:
  Bus Creator : BusCreator  Inputs=6
  Geschwindigkeitsregler : Subsystem
  Gierdämpfer : Subsystem
  Headingregler : Subsystem
  Höhenregler : Subsystem
  current waypoint location : Subsystem
  plane location : Subsystem
  waypoint rached : Subsystem
  waypoint reached : Outport
  Throttle [0-1] : Outport  Port=2
  delta_eta [deg] : Outport  Port=3
  aileron [deg] : Outport  Port=4
  heading error [rad] : Outport  Port=5
  distance to waypoint [m] : Outport  Port=6
  Koordinatenzeugs : Outport  Port=7
  wires:
  plane location/1(x_aircraft [m]) -> [x_aircraft_m]
  plane location/2(y_aircraft [m]) -> [y_aircraft_m]
  current waypoint location/2(y_waypoit [m]) -> [y_waypoint_m]
  current waypoint location/1(x_waypoint [m]) -> [x_waypoint_m]
  [x_aircraft_m] -> waypoint rached/1(x_aircraft [m])
  [y_aircraft_m] -> waypoint rached/2(y_aircraft [m])
  [x_waypoint_m] -> waypoint rached/3(x_waypoint [m])
  [y_waypoint_m] -> waypoint rached/4(y_waypoit [m])
  waypoint rached/1(waypoint reached) -> waypoint reached/1
  Vehicle States/1 -> [Vehicle_States]
  Telemetry Data/1 -> [Telemetry_Data]
  [Vehicle_States] -> plane location/1(Vehicle States)
  [Telemetry_Data] -> current waypoint location/2(Telemetry Data)
  [Vehicle_States] -> current waypoint location/1(Vehicle States)
  plane location/3(z_aircraft [m]) -> [z_aircraft_m]
  current waypoint location/3(z_waypoint [m]) -> [z_waypoint_m]
  [z_aircraft_m] -> Höhenregler/1(z_aircraft [m])
  [z_waypoint_m] -> Höhenregler/2(z_waypoint [m])
  [Vehicle_States] -> Höhenregler/3(Vehicel States)
  [Vehicle_States] -> Geschwindigkeitsregler/1(Vehicle States)
  [Telemetry_Data] -> Geschwindigkeitsregler/2(Telemetry Data)
  Geschwindigkeitsregler/1(Throttle [0-1]) -> Throttle [0-1]/1
  Höhenregler/1(delta_eta [deg]) -> delta_eta [deg]/1
  [Vehicle_States] -> Gierdämpfer/1(Vehicle States)
  [y_waypoint_m] -> Headingregler/4(y waypoint [m])
  [x_waypoint_m] -> Headingregler/3(x waypoint [m])
  [y_aircraft_m] -> Headingregler/2(y aircraft [m])
  [x_aircraft_m] -> Headingregler/1(x aircraft [m])
  [Vehicle_States] -> Headingregler/5(Vehicle States)
  Headingregler/1(aileronausschlag) -> aileron [deg]/1
  Headingregler/2(heading error) -> heading error [rad]/1
  waypoint rached/2(distance to waypoint [m]) -> distance to waypoint [m]/1
  [x_aircraft_m] -> Bus Creator/1  "x_aircraft_m"
  [y_aircraft_m] -> Bus Creator/2  "y_aircraft_m"
  [x_waypoint_m] -> Bus Creator/3  "x_waypoint_m"
  [y_waypoint_m] -> Bus Creator/4  "y_waypoint_m"
  [waypoint_breitengrad_rad] -> Bus Creator/5  "waypoint_breitengrad_rad"
  [waypoint_laengengrad_rad] -> Bus Creator/6  "waypoint_laengengrad_rad"
  current waypoint location/4(waypoint_breitengrad_rad) -> [waypoint_breitengrad_rad]
  current waypoint location/5(waypoint_laengengrad_rad) -> [waypoint_laengengrad_rad]
  Bus Creator/1 -> Koordinatenzeugs/1

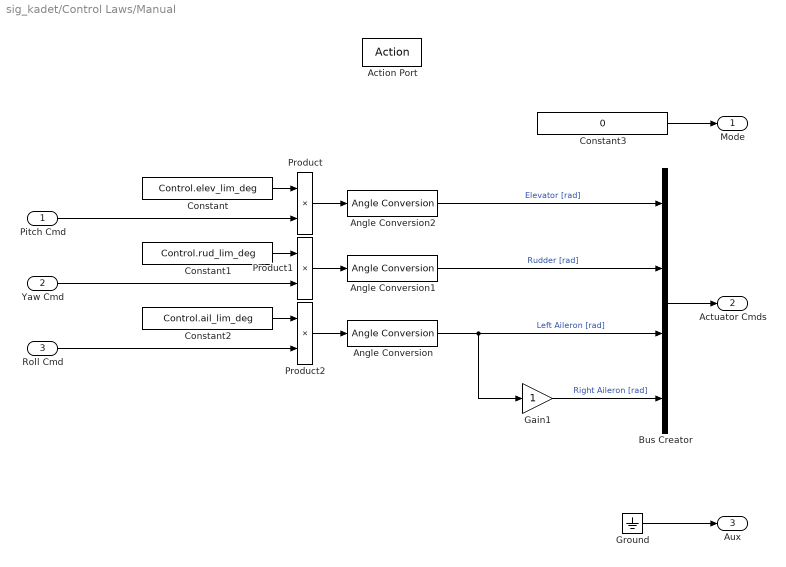
== system sig_kadet/Control Laws/Manual ==
  Pitch Cmd : Inport
  Yaw Cmd : Inport  Port=2
  Roll Cmd : Inport  Port=3
  Action Port : ActionPort  InitializeStates=reset  ActionPortLabel=default:
  Angle Conversion : aerolibconvert2/Angle Conversion  IU=deg  OU=rad
  Angle Conversion1 : aerolibconvert2/Angle Conversion  IU=deg  OU=rad
  Angle Conversion2 : aerolibconvert2/Angle Conversion  IU=deg  OU=rad
  Bus Creator : BusCreator  Inputs=4
  Constant : Constant  Value=Control.elev_lim_deg  OutDataTypeStr=single
  Constant1 : Constant  Value=Control.rud_lim_deg  OutDataTypeStr=single
  Constant2 : Constant  Value=Control.ail_lim_deg  OutDataTypeStr=single
  Constant3 : Constant  Value=0  OutDataTypeStr=int8
  Gain1 : Gain  OutDataTypeStr=single
  Ground : Ground
  Product : Product  OutDataTypeStr=single
  Product1 : Product  OutDataTypeStr=single
  Product2 : Product  OutDataTypeStr=single
  Mode : Outport
  Actuator Cmds : Outport  Port=2
  Aux : Outport  Port=3
  wires:
  Angle Conversion1/1 -> Bus Creator/2  "Rudder [rad]"
  Product2/1 -> Angle Conversion/1
  Yaw Cmd/1 -> Product1/2
  Roll Cmd/1 -> Product2/2
  Angle Conversion/1 -> Gain1/1, Bus Creator/3  "Left Aileron [rad]"
  Product1/1 -> Angle Conversion1/1
  Pitch Cmd/1 -> Product/2
  Gain1/1 -> Bus Creator/4  "Right Aileron [rad]"
  Constant1/1 -> Product1/1
  Angle Conversion2/1 -> Bus Creator/1  "Elevator [rad]"
  Product/1 -> Angle Conversion2/1
  Constant/1 -> Product/1
  Constant2/1 -> Product2/1
  Bus Creator/1 -> Actuator Cmds/1
  Constant3/1 -> Mode/1
  Ground/1 -> Aux/1

== system sig_kadet/Control Laws/Manual Throttle ==
  Throttle Cmd : Inport
  Yaw Cmd : Inport  Port=2
  Action Port : ActionPort  InitializeStates=reset  ActionPortLabel=default:
  Data Type Conversion : DataTypeConversion  OutDataTypeStr=single  SaturateOnIntegerOverflow=off  RndMeth=Floor
  Gain : Gain  OutDataTypeStr=single
  Gain1 : Gain  Gain=0.2  OutDataTypeStr=single
  Saturation : Saturate  UpperLimit=1  LowerLimit=0
  Sum : Sum  Inputs=|++
  Throttle [0 - 1] : Outport
  wires:
  Saturation/1 -> Data Type Conversion/1  "Throttle [0 - 1]"
  Throttle Cmd/1 -> Gain/1
  Yaw Cmd/1 -> Gain1/1
  Gain1/1 -> Sum/2  "Yaw [-0.2 - 0.2]"
  Gain/1 -> Sum/1  "Throttle [0 - 1]"
  Sum/1 -> Saturation/1
  Data Type Conversion/1 -> Throttle [0 - 1]/1

== system sig_kadet/Sensor Processing/Analog Input Mapping ==
  note: FMU-R v2.x has 8 channels of analog input
      | data from 0 - 3.3V. The measured voltage
      | is available from the ADC data input, this is
      | an opportunity to map the voltage data to
      | engineering units (i.e. control surface position,
      | acceleration, etc) for logging and use elsewhere
      | in the VMS.
  ADC : Inport
  Bus Creator : BusCreator  Inputs=1  OutDataTypeStr=Bus: AnalogData
  Bus Selector : BusSelector  OutputSignals=volt
  Gain : Gain  Gain=0
  Analog Data : Outport
  wires:
  ADC/1 -> Bus Selector/1
  Bus Selector/1 -> Gain/1  "<volt>"
  Bus Creator/1 -> Analog Data/1
  Gain/1 -> Bus Creator/1

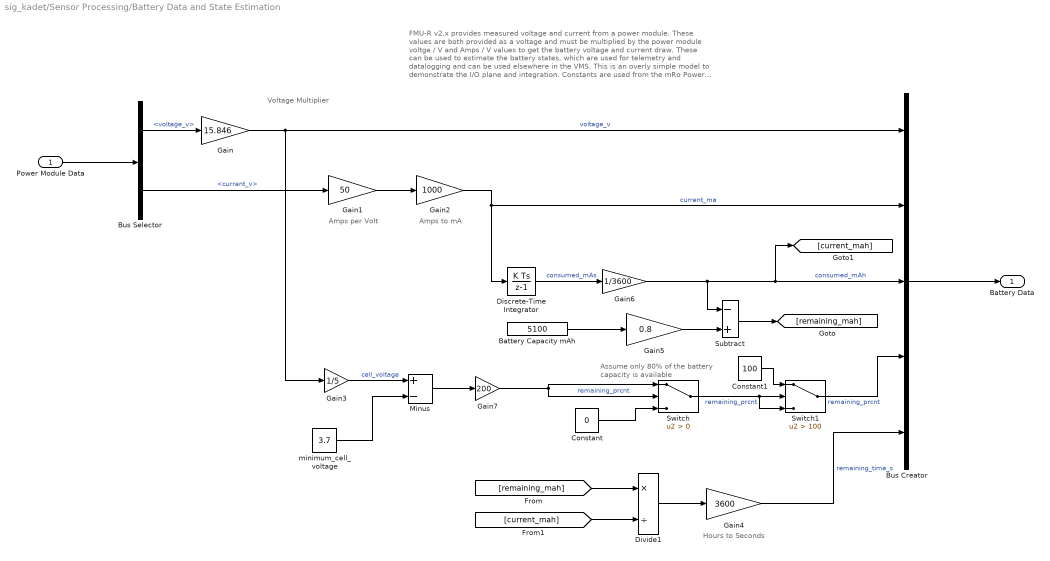
== system sig_kadet/Sensor Processing/Battery Data and State Estimation ==
  note: Assume only 80% of
      | the battery capacity is available
  note: Hours to Seconds
  note: Amps to mA
  note: Amps per Volt
  note: Voltage Multiplier
  note: FMU-R v2.x provides measured voltage and current from a power module.
      | These values are both provided as a voltage and must be multiplied by the
      | power module voltge / V and Amps / V values to get the battery voltage
      | and current draw. These can be used to estimate the battery states, which
      | are used for telemetry and datalogging and can be used elsewhere in the VMS.
      |
      | This is an overly simple model to demonstrate the I/O plane and integration.
      | Constants are used from the mRo Power Zero module.
  Power Module Data : Inport
  Battery Capacity mAh : Constant  Value=5100  OutDataTypeStr=single
  Bus Creator : BusCreator  Inputs=5  OutDataTypeStr=Bus: BatteryData
  Bus Selector : BusSelector  OutputSignals=voltage_v,current_v
  Constant : Constant  Value=0
  Constant1 : Constant  Value=100
  Discrete-Time Integrator : DiscreteIntegrator  SampleTime=framePeriod_s  ICPrevOutput=DiscIntNeverNeededParam  ICPrevScaledInput=DiscIntNeverNeededParam
  Divide1 : Product  Inputs=*/
  Gain : Gain  Gain=15.846
  Gain1 : Gain  Gain=50
  Gain2 : Gain  Gain=1000
  Gain3 : Gain  Gain=1/5
  Gain4 : Gain  Gain=3600
  Gain5 : Gain  Gain=0.8
  Gain6 : Gain  Gain=1/3600
  Gain7 : Gain  Gain=200
  Minus : Sum  Inputs=+-
  Subtract : Sum  Inputs=-+
  Switch : Switch  Criteria=u2 > Threshold  OutDataTypeStr=single  SaturateOnIntegerOverflow=off  InputSameDT=off
  Switch1 : Switch  Criteria=u2 > Threshold  Threshold=100  OutDataTypeStr=single  SaturateOnIntegerOverflow=off  InputSameDT=off
  minimum_cell_voltage : Constant  Value=3.7
  Battery Data : Outport
  wires:
  Power Module Data/1 -> Bus Selector/1
  Bus Selector/1 -> Gain/1  "<voltage_v>"
  Bus Selector/2 -> Gain1/1  "<current_v>"
  Gain1/1 -> Gain2/1
  Gain2/1 -> Discrete-Time Integrator/1, Bus Creator/2  "current_ma"
  Gain/1 -> Bus Creator/1, Gain3/1  "voltage_v"
  Discrete-Time Integrator/1 -> Gain6/1  "consumed_mAs"
  Bus Creator/1 -> Battery Data/1
  Subtract/1 -> [remaining_mah]
  Gain5/1 -> Subtract/2
  [remaining_mah] -> Divide1/1
  [current_mah] -> Divide1/2
  Gain4/1 -> Bus Creator/5  "remaining_time_s"
  Divide1/1 -> Gain4/1
  Battery Capacity mAh/1 -> Gain5/1
  Gain6/1 -> Subtract/1, [current_mah], Bus Creator/3  "consumed_mAh"
  Gain3/1 -> Minus/1  "cell_voltage"
  minimum_cell_voltage/1 -> Minus/2
  Minus/1 -> Gain7/1
  Gain7/1 -> Switch/2, Switch/1  "remaining_prcnt"
  Constant/1 -> Switch/3
  Switch1/1 -> Bus Creator/4  "remaining_prcnt"
  Switch/1 -> Switch1/3, Switch1/2  "remaining_prcnt"
  Constant1/1 -> Switch1/1

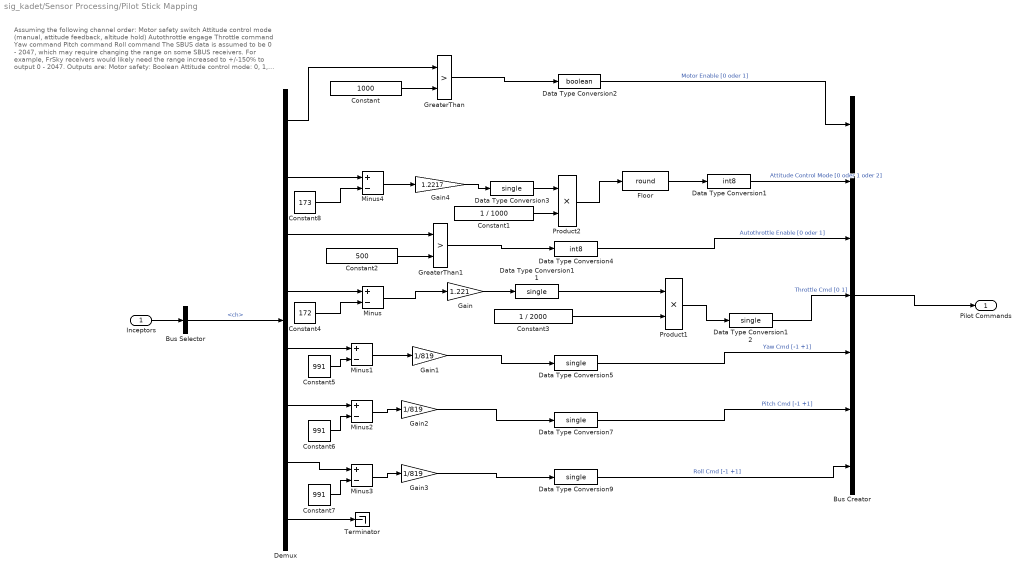
== system sig_kadet/Sensor Processing/Pilot Stick Mapping ==
  note: Assuming the following channel order:
      | Motor safety switch
      | Attitude control mode (manual, attitude feedback, altitude hold)
      | Autothrottle engage
      | Throttle command
      | Yaw command
      | Pitch command
      | Roll command
      |
      | The SBUS data is assumed to be 0 - 2047, which may require changing the
      | range on some SBUS receivers. For example, FrSky receivers would
      | likely need the range increased to +/-150% to output 0 - 2047.
      |
      | Outputs are:
      | Motor safety: Boolean
      | Attitude control mode: 0, 1, 2 integer
      | Autothrottle engage: Boolean
      | Throttle command: 0 to 1 single
      | Yaw command: -1 to +1 single
      | Pitch command: -1 to +1 single
      | Roll command: -1 to +1 single
  Inceptors : Inport
  Bus Creator : BusCreator  Inputs=7
  Bus Selector : BusSelector  OutputSignals=ch
  Constant : Constant  Value=1000
  Constant1 : Constant  Value=1 / 1000  OutDataTypeStr=single
  Constant2 : Constant  Value=500  OutDataTypeStr=int16
  Constant3 : Constant  Value=1 / 2000  OutDataTypeStr=single
  Constant4 : Constant  Value=172
  Constant5 : Constant  Value=991
  Constant6 : Constant  Value=991
  Constant7 : Constant  Value=991
  Constant8 : Constant  Value=173
  Data Type Conversion1 : DataTypeConversion  OutDataTypeStr=int8  SaturateOnIntegerOverflow=off  RndMeth=Floor
  Data Type Conversion{3,5,7,9,11..12} (6 alike) : DataTypeConversion  OutDataTypeStr=single  SaturateOnIntegerOverflow=off  RndMeth=Floor
  Data Type Conversion2 : DataTypeConversion  OutDataTypeStr=boolean  SaturateOnIntegerOverflow=off  RndMeth=Floor
  Data Type Conversion4 : DataTypeConversion  OutDataTypeStr=int8  SaturateOnIntegerOverflow=off  RndMeth=Floor
  Demux : Demux  Outputs=[1 1 1 1 1 1 1 9]
  Floor : Rounding  Operator=round
  Gain : Gain  Gain=1.221
  Gain1 : Gain  Gain=1/819
  Gain2 : Gain  Gain=1/819
  Gain3 : Gain  Gain=1/819
  Gain4 : Gain  Gain=1.2217
  GreaterThan : RelationalOperator  Operator=>  OutDataTypeStr=boolean  RndMeth=Simplest  InputSameDT=off
  GreaterThan1 : RelationalOperator  Operator=>  OutDataTypeStr=boolean  RndMeth=Simplest  InputSameDT=off
  Minus{,1..4} (5 alike) : Sum  Inputs=+-
  Product1 : Product
  Product2 : Product
  Terminator : Terminator
  Pilot Commands : Outport
  wires:
  Inceptors/1 -> Bus Selector/1
  Bus Selector/1 -> Demux/1  "<ch>"
  Constant/1 -> GreaterThan/2
  Demux/1 -> GreaterThan/1
  GreaterThan/1 -> Data Type Conversion2/1
  Product2/1 -> Floor/1
  Demux/3 -> GreaterThan1/1
  Constant2/1 -> GreaterThan1/2
  GreaterThan1/1 -> Data Type Conversion4/1
  Floor/1 -> Data Type Conversion1/1
  Gain2/1 -> Data Type Conversion7/1
  Gain3/1 -> Data Type Conversion9/1
  Demux/8 -> Terminator/1
  Data Type Conversion11/1 -> Product1/1
  Constant3/1 -> Product1/2
  Demux/4 -> Minus/1
  Product1/1 -> Data Type Conversion12/1
  Bus Creator/1 -> Pilot Commands/1
  Data Type Conversion2/1 -> Bus Creator/1  "Motor Enable [0 oder 1]"
  Data Type Conversion1/1 -> Bus Creator/2  "Attitude Control Mode [0 oder 1 oder 2]"
  Data Type Conversion4/1 -> Bus Creator/3  "Autothrottle Enable [0 oder 1]"
  Data Type Conversion12/1 -> Bus Creator/4  "Throttle Cmd [0 1]"
  Data Type Conversion5/1 -> Bus Creator/5  "Yaw Cmd [-1 +1]"
  Data Type Conversion7/1 -> Bus Creator/6  "Pitch Cmd [-1 +1]"
  Data Type Conversion9/1 -> Bus Creator/7  "Roll Cmd [-1 +1]"
  Minus/1 -> Gain/1
  Constant4/1 -> Minus/2
  Gain/1 -> Data Type Conversion11/1
  Demux/5 -> Minus1/1
  Constant5/1 -> Minus1/2
  Gain1/1 -> Data Type Conversion5/1
  Minus1/1 -> Gain1/1
  Constant6/1 -> Minus2/2
  Demux/6 -> Minus2/1
  Minus2/1 -> Gain2/1
  Minus3/1 -> Gain3/1
  Constant7/1 -> Minus3/2
  Demux/7 -> Minus3/1
  Demux/2 -> Minus4/1
  Constant8/1 -> Minus4/2
  Minus4/1 -> Gain4/1
  Data Type Conversion3/1 -> Product2/1
  Constant1/1 -> Product2/2
  Gain4/1 -> Data Type Conversion3/1

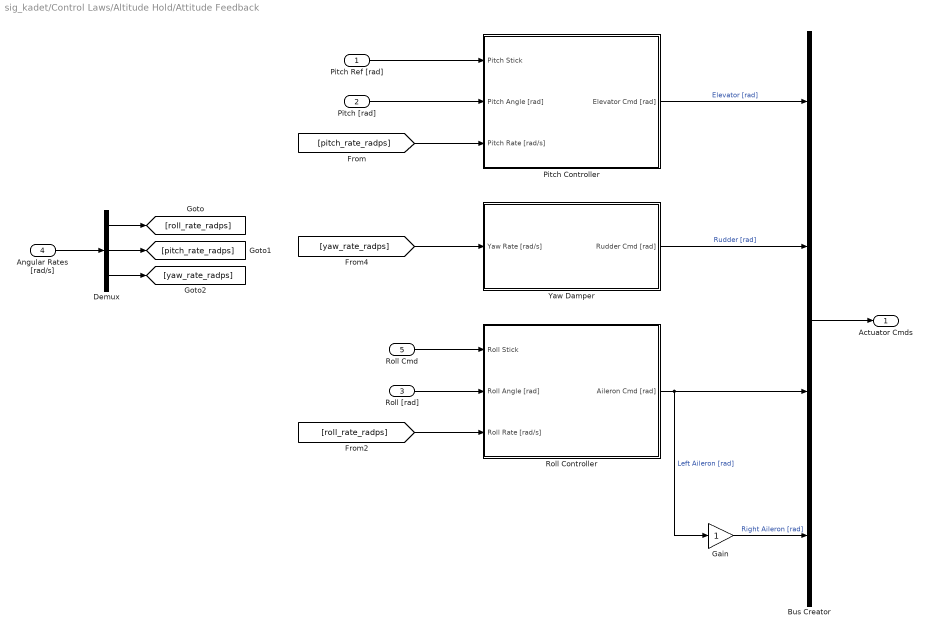
== system sig_kadet/Control Laws/Altitude Hold/Attitude Feedback ==
  Pitch Ref [rad] : Inport
  Pitch [rad] : Inport  Port=2
  Roll [rad] : Inport  Port=3
  Angular Rates [rad/s] : Inport  Port=4
  Roll Cmd : Inport  Port=5
  Bus Creator : BusCreator  Inputs=4
  Demux : Demux  Outputs=3
  Gain : Gain
  Pitch Controller : Subsystem
  Roll Controller : Subsystem
  Yaw Damper : Subsystem
  Actuator Cmds : Outport
  wires:
  Pitch [rad]/1 -> Pitch Controller/2(Pitch Angle [rad])
  Angular Rates [rad/s]/1 -> Demux/1
  Demux/1 -> [roll_rate_radps]
  Demux/3 -> [yaw_rate_radps]
  Demux/2 -> [pitch_rate_radps]
  [pitch_rate_radps] -> Pitch Controller/3(Pitch Rate [rad/s])
  Pitch Ref [rad]/1 -> Pitch Controller/1(Pitch Stick)
  Pitch Controller/1(Elevator Cmd [rad]) -> Bus Creator/1  "Elevator [rad]"
  Bus Creator/1 -> Actuator Cmds/1
  Gain/1 -> Bus Creator/4  "Right Aileron [rad]"
  Roll Controller/1(Aileron Cmd [rad]) -> Gain/1, Bus Creator/3  "Left Aileron [rad]"
  Yaw Damper/1(Rudder Cmd [rad]) -> Bus Creator/2  "Rudder [rad]"
  Roll [rad]/1 -> Roll Controller/2(Roll Angle [rad])
  [roll_rate_radps] -> Roll Controller/3(Roll Rate [rad/s])
  Roll Cmd/1 -> Roll Controller/1(Roll Stick)
  [yaw_rate_radps] -> Yaw Damper/1(Yaw Rate [rad/s])

== system sig_kadet/Control Laws/Altitude Hold/Latch Initial Value ==
  Value : Inport
  Constant : Constant  Value=0
  Switch : Switch  Criteria=u2 > Threshold  SaturateOnIntegerOverflow=off  InputSameDT=off
  Unit Delay : UnitDelay  SampleTime=-1  HasFrameUpgradeWarning=on
  Unit Delay1 : UnitDelay  InitialCondition=1  SampleTime=-1  HasFrameUpgradeWarning=on
  Latched Value : Outport
  wires:
  Unit Delay/1 -> Switch/3
  Value/1 -> Switch/1
  Constant/1 -> Unit Delay1/1
  Unit Delay1/1 -> Switch/2
  Switch/1 -> Unit Delay/1, Latched Value/1
